simulink model "back_left_leg_assembly"  (R2023b)
settings: Solver=VariableStepAuto  StartTime=0.0  StopTime=10.0  RelTol=1e-3  AbsTol=1e-3  EnableMultiTasking=on
undefined symbols (not defined in the file): robot_conversions, robot_joints, robot_weights, X, Y, Z
libraries: sm_lib x17, nesl_utility x7, cstblocks x6, simulink x3, simulink_extras x3
settings Model: Creator=ivano  LastModifiedBy=ivano
settings SolverCC: AutoScaleAbsTol=off  AlgebraicLoopSolver=TrustRegion  MaxZcPerStep=1
settings DataIOCC: LimitDataPoints=on  MaxDataPoints=10000
settings OptimizationCC: ReuseModelBlockBuffer=off  LifeSpan=inf
settings DebuggingCC: UnconnectedInputMsg=warning  UnconnectedOutputMsg=warning  UnconnectedLineMsg=warning  AllowSymbolicDim=off  SubsystemReferenceDiagnosticForUnitTest=warning  SFUnexpectedBacktrackingDiag=warning  SFNoUnconditionalDefaultTransitionDiag=warning  SFExecutionAtInitializationDiag=none  ArithmeticOperatorsInVariantConditions=warning
settings ModelReferenceCC: EnableRefExpFcnMdlSchedulingChecks=on
settings SFSimCC: SimUseLocalCustomCode=off  CustomCodeUndefinedFunction=UseInterfaceOnly
settings RTWCC: RTWUseLocalCustomCode=off  DLArmComputeVersion=19.05
settings CodeAppCC: StateflowObjectComments=on
settings GRTTargetCC: TargetLangStandard=C89/C90 (ANSI)
settings ConfigComp: CovMetricSettings=dw  CovSaveCumulativeToWorkspaceVar=on  CovSaveSingleToWorkspaceVar=on  CovExternalEMLEnable=off  CovSFcnEnable=off
settings SimscapeCC: SimscapeLogType=all  SimscapeLogSimulationStatistics=on  SimscapeLogDataHistory=10000

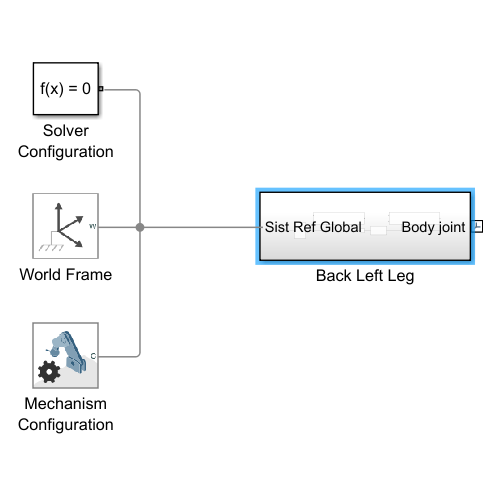
[thumbnail: Simulink's stored preview of the top-level diagram]
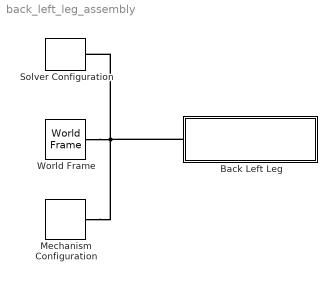
== system back_left_leg_assembly ==
  Back Left Leg : Subsystem
  Mechanism Configuration : sm_lib/Utilities/Mechanism Configuration  UniformGravity=Constant  GravityVector=[0 0 -9.80665]  GravityVectorUnits=m/s^2  LinearizationDelta=0.001  JointModeTransitionNonlinearIterations=2
  Solver Configuration : nesl_utility/Solver Configuration  PhysicalDomain=network_engine_domain  SubClassName=solver  LeftPortType=input  RightPortType=generic  Tones=[]  Harmonics=[]  SimulateNoise=off  Profile=off  UseLocalSampling=off  EnableSwitchedLinearOptims=on  FrequencyDomain=off  UseCCode=off  RelTol=0.001  AbsTol=1e-06  MinStep=1e-09  ToWorkspace=off  RevertToSquareIcSolve=off  NumHomotopyIterations=100  PhasorMode=off  PhasorModeNumHarmonics=1  ConsistencySolver=NEWTON_XTOL_AFTER_FTOL  IndexReductionMethod=DerivativeReplacement  DoDC=off  ResidualTolerance=1e-09  ConsistencyTolSource=GLOBAL  ConsistencyAbsTol=0.001  ConsistencyRelTol=0.001  ConsistencyTolFactor=0.001  UseLocalSolver=off  LocalSolverChoice=NE_BACKWARD_EULER_ADVANCER  ResolveIndetEquations=on  FunctionEvalNumThread=1  LocalSolverSampleTime=0.001  DoFixedCost=off  MaxNonlinIter=3  MaxModeIter=2  ComputeImpulses=off  ImpulseIterations=2  LinearAlgebra=Sparse  LinearAlgebraNumThread=0  EquationFormulation=NE_TIME_EF  DelaysMemoryBudget=1024  AutomaticFiltering=on  FilteringTimeConstant=0.001  PartitionStorageMethod=AS_NEEDED  PartitionMemoryBudget=1024  PartitionMethod=FAST  MultibodyUseLocalSolver=off  MultibodyLocalSolverChoice=ODE1  MultibodyLocalSolverSampleTime=0.001
  World Frame : sm_lib/Frames and Transforms/World Frame
  connections:
  World Frame/RConn1 -- Mechanism Configuration/RConn1 -- Back Left Leg/LConn1 -- Solver Configuration/RConn1

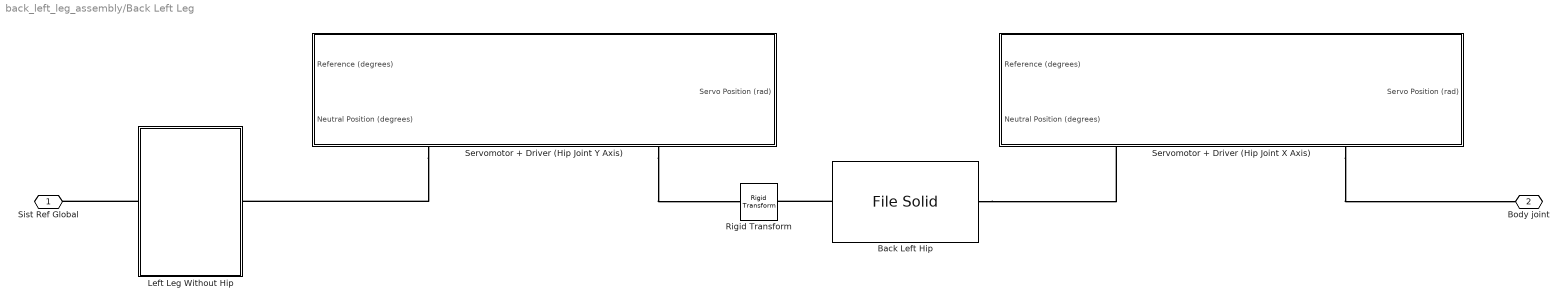
== system back_left_leg_assembly/Back Left Leg ==
  Back Left Hip : sm_lib/Body Elements/File Solid  ExtGeomFileName=..\3D Models\Hip\STEP Simscape Models\hip_bl.step  UnitType=FromFile  ExtGeomFileUnits=m  StepReaderType=HEX  ExportConvexHullGeometry=off  InertiaType=CalculateFromGeometry  Mass=robot_weights.hip  MassUnits=g  CenterOfMass=[0 0 0]  CenterOfMassUnits=m  MomentsOfInertia=[1 1 1]  MomentsOfInertiaUnits=kg*m^2  ProductsOfInertia=[0 0 0]  ProductsOfInertiaUnits=kg*m^2  BasedOnType=Mass  Density=1000  DensityUnits=kg/m^3  DoExposeReferenceFrame=off  SerializedFrames=<Frames><Frame><Id>Frame1</Id><Value><Name>Femur_joint</Name><Origin><Source>GeometricFeature</Source><FeatureName>circular curve 60</FeatureName></Origin><PrimaryAxis><DefinedDirection>+Z</DefinedDirection><Source>ReferenceFrame</Source><SourceDirection>+Z</SourceDirection><FeatureName></FeatureName></PrimaryAxis><SecondaryAxis><DefinedDirection>+X</DefinedDirection><Source>ReferenceFrame</Source><SourceDirection>+X</SourceDirection><FeatureName></FeatureName></SecondaryAxis></Value></Frame><Frame><Id>Frame2</Id><Value><Name>Body_joint</Name><Origin><Source>GeometricFeature</Source><FeatureName>circular curve 72</FeatureName></Origin><PrimaryAxis><DefinedDirection>+Z</DefinedDirection><Source>ReferenceFrame</Source><SourceDirection>+Z</SourceDirection><FeatureName></FeatureName></PrimaryAxis><SecondaryAxis><DefinedDirection>+X</DefinedDirection><Source>ReferenceFrame</Source><SourceDirection>+X</SourceDirection><FeatureName></FeatureName></SecondaryAxis></Value></Frame></Frames>  GraphicType=FromGeometry  MarkerShape=Sphere  MarkerSize=10  GraphicVisPropType=SimpleVisualProperties  GraphicDiffuseColor=[0.5 0.5 0.5]  GraphicSpecularColor=[0.5 0.5 0.5 1.0]  GraphicAmbientColor=[0.15 0.15 0.15 1.0]  GraphicEmissiveColor=[0.0 0.0 0.0 1.0]  GraphicShininess=75  GraphicOpacity=1.0
  Left Leg Without Hip : Subsystem
  Rigid Transform : sm_lib/Frames and Transforms/Rigid Transform  TranslationMethod=Cartesian  TranslationStandardOffset=0  TranslationStandardOffsetUnits=m  TranslationStandardAxis=+Z  TranslationCartesianOffset=[0 9.477 0]  TranslationCartesianOffsetUnits=mm  TranslationROffset=0  TranslationROffsetUnits=m  TranslationZOffset=0  TranslationZOffsetUnits=m  TranslationThetaOffset=0  TranslationThetaOffsetUnits=deg  RotationMethod=None  RotationAngleUnits=deg  RotationStandardAxis=+Z  RotationAngle=0.0  RotationArbitraryAxis=[0 0 1]  FollAlignAxisA=+X  BaseAlignAxisA=+Y  FollAlignAxisB=+Y  BaseAlignAxisB=+Z  RotationSequenceAxes=FollowerAxes  RotationSequence=XYX  RotationSequenceAngles=[0 0 0]  RotationSequenceAnglesUnits=deg  RotationMatrix=[1 0 0; 0 1 0; 0 0 1]  Quaternion=[1 0 0 0]
  Servomotor + Driver (Hip Joint X Axis) : Subsystem
      settings: PortSchema="{\"entries\":[{\"content\":{\"sides\":[{\"content\":{\"connectorIds\":[\"In1\",\"In2\"]},\"type\":\"ConnectorPlacement.EquallySpacedRectSide\",\"uuid\":\"34aed934-2639-4a00-aaee-cf3027466446\"},{\"content\":{\"connectorIds\":[\"Out1\"],\"side\":\"RIGHT\"},\"type\":\"ConnectorPlacement.EquallySpacedRectSide\",\"uuid\":\"6801890d-3466-4e37-90e8-6d1471e5b2c4\"},{\"content\":{\"side\":\"TOP\"},\"type\":\"ConnectorPlacement.EquallySpacedRectSide\",\"uuid\":\"bc3191aa-eca4-4e32-9fcf-8d5b7059b0b6\"},{\"content\":{\"connectorIds\":[\"RConn1\",\"RConn2\"],\"side\":\"BOTTOM\"},\"type\":\"ConnectorPlacement.EquallySpacedRectSide\",\"uuid\":\"867f09f9-bc2c-4353-bf05-5e7fc6d76fc7\"}]},\"type\":\"ConnectorPlacement.EquallySpacedConnector\",\"uuid\":\"7616468a-464c-41b8-bfd7-188201b948eb\"}],\"packageUris\":[\"http://schema.mathworks.com/mf0/Connector/R2020b\"],\"version\":\"1.0\"}"
  Servomotor + Driver (Hip Joint Y Axis) : Subsystem
      settings: PortSchema="{\"entries\":[{\"content\":{\"sides\":[{\"content\":{\"connectorIds\":[\"In1\",\"In2\"]},\"type\":\"ConnectorPlacement.EquallySpacedRectSide\",\"uuid\":\"34aed934-2639-4a00-aaee-cf3027466446\"},{\"content\":{\"connectorIds\":[\"Out1\"],\"side\":\"RIGHT\"},\"type\":\"ConnectorPlacement.EquallySpacedRectSide\",\"uuid\":\"6801890d-3466-4e37-90e8-6d1471e5b2c4\"},{\"content\":{\"side\":\"TOP\"},\"type\":\"ConnectorPlacement.EquallySpacedRectSide\",\"uuid\":\"bc3191aa-eca4-4e32-9fcf-8d5b7059b0b6\"},{\"content\":{\"connectorIds\":[\"RConn1\",\"RConn2\"],\"side\":\"BOTTOM\"},\"type\":\"ConnectorPlacement.EquallySpacedRectSide\",\"uuid\":\"867f09f9-bc2c-4353-bf05-5e7fc6d76fc7\"}]},\"type\":\"ConnectorPlacement.EquallySpacedConnector\",\"uuid\":\"7616468a-464c-41b8-bfd7-188201b948eb\"}],\"packageUris\":[\"http://schema.mathworks.com/mf0/Connector/R2020b\"],\"version\":\"1.0\"}"
  Sist Ref Global : PMIOPort  Side=Left
  Body joint : PMIOPort  Port=2  Side=Right
  connections:
  Servomotor + Driver (Hip Joint Y Axis)/RConn2 -- Rigid Transform/RConn1
  Back Left Hip/LConn1 -- Rigid Transform/LConn1
  Servomotor + Driver (Hip Joint Y Axis)/RConn1 -- Left Leg Without Hip/RConn1
  Left Leg Without Hip/LConn1 -- Sist Ref Global/RConn1
  Back Left Hip/RConn1 -- Servomotor + Driver (Hip Joint X Axis)/RConn1
  Servomotor + Driver (Hip Joint X Axis)/RConn2 -- Body joint/RConn1

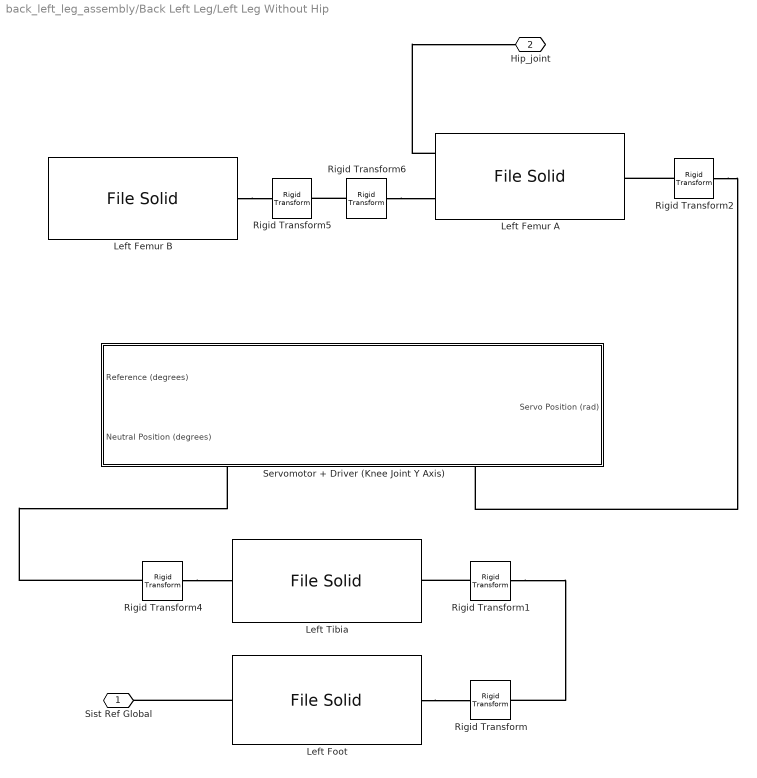
== system back_left_leg_assembly/Back Left Leg/Left Leg Without Hip ==
  Left Femur A : sm_lib/Body Elements/File Solid  ExtGeomFileName=..\3D Models\Femur\STEP Simscape Models\femur_l_a.step  UnitType=FromFile  ExtGeomFileUnits=m  StepReaderType=HEX  ExportConvexHullGeometry=off  InertiaType=CalculateFromGeometry  Mass=robot_weights.femur_a  MassUnits=g  CenterOfMass=[0 0 0]  CenterOfMassUnits=m  MomentsOfInertia=[1 1 1]  MomentsOfInertiaUnits=kg*m^2  ProductsOfInertia=[0 0 0]  ProductsOfInertiaUnits=kg*m^2  BasedOnType=Mass  Density=1000  DensityUnits=kg/m^3  DoExposeReferenceFrame=off  SerializedFrames=<Frames><Frame><Id>Frame1</Id><Value><Name>Hip_joint</Name><Origin><Source>GeometricFeature</Source><FeatureName>circular curve 110</FeatureName></Origin><PrimaryAxis><DefinedDirection>+Z</DefinedDirection><Source>ReferenceFrame</Source><SourceDirection>+Z</SourceDirection><FeatureName></FeatureName></PrimaryAxis><SecondaryAxis><DefinedDirection>+X</DefinedDirection><Source>ReferenceFrame</Source><SourceDirection>+X</SourceDirection><FeatureName></FeatureName></SecondaryAxis></Value></Frame><Frame><Id>Frame2</Id><Value><Name>Tibia_joint</Name><Origin><Source>GeometricFeature</Source><FeatureName>circular curve 126</FeatureName></Origin><PrimaryAxis><DefinedDirection>+Z</DefinedDirection><Source>ReferenceFrame</Source><SourceDirection>+Z</SourceDirection><FeatureName></FeatureName></PrimaryAxis><SecondaryAxis><DefinedDirection>+X</DefinedDirection><Source>ReferenceFrame</Source><SourceDirection>+X</SourceDirection><FeatureName></FeatureName></SecondaryAxis></Value></Frame><Frame><Id>Frame3</Id><Value><Name>Femur_B_joint</Name><Origin><Source>GeometricFeature</Source><FeatureName>circular curve 10</FeatureName></Origin><PrimaryAxis><DefinedDirection>+Z</DefinedDirection><Source>ReferenceFrame</Source><SourceDirection>+Z</SourceDirection><FeatureName></FeatureName></PrimaryAxis><SecondaryAxis><DefinedDirection>+X</DefinedDirection><Source>ReferenceFrame</Source><SourceDirection>+X</SourceDirection><FeatureName></FeatureName></SecondaryAxis></Value></Frame></Frames>  GraphicType=FromGeometry  MarkerShape=Sphere  MarkerSize=10  GraphicVisPropType=SimpleVisualProperties  GraphicDiffuseColor=[0.5 0.5 0.5]  GraphicSpecularColor=[0.5 0.5 0.5 1.0]  GraphicAmbientColor=[0.15 0.15 0.15 1.0]  GraphicEmissiveColor=[0.0 0.0 0.0 1.0]  GraphicShininess=75  GraphicOpacity=1.0
  Left Femur B : sm_lib/Body Elements/File Solid  ExtGeomFileName=..\3D Models\Femur\STEP Simscape Models\femur_l_b.step  UnitType=FromFile  ExtGeomFileUnits=m  StepReaderType=HEX  ExportConvexHullGeometry=off  InertiaType=CalculateFromGeometry  Mass=robot_weights.femur_b  MassUnits=g  CenterOfMass=[0 0 0]  CenterOfMassUnits=m  MomentsOfInertia=[1 1 1]  MomentsOfInertiaUnits=kg*m^2  ProductsOfInertia=[0 0 0]  ProductsOfInertiaUnits=kg*m^2  BasedOnType=Mass  Density=1000  DensityUnits=kg/m^3  DoExposeReferenceFrame=off  SerializedFrames=<Frames><Frame><Id>Frame1</Id><Value><Name>Femur_A_joint</Name><Origin><Source>GeometricFeature</Source><FeatureName>circular curve 235</FeatureName></Origin><PrimaryAxis><DefinedDirection>+Z</DefinedDirection><Source>ReferenceFrame</Source><SourceDirection>+Z</SourceDirection><FeatureName></FeatureName></PrimaryAxis><SecondaryAxis><DefinedDirection>+X</DefinedDirection><Source>ReferenceFrame</Source><SourceDirection>+X</SourceDirection><FeatureName></FeatureName></SecondaryAxis></Value></Frame></Frames>  GraphicType=FromGeometry  MarkerShape=Sphere  MarkerSize=10  GraphicVisPropType=SimpleVisualProperties  GraphicDiffuseColor=[0.5 0.5 0.5]  GraphicSpecularColor=[0.5 0.5 0.5 1.0]  GraphicAmbientColor=[0.15 0.15 0.15 1.0]  GraphicEmissiveColor=[0.0 0.0 0.0 1.0]  GraphicShininess=75  GraphicOpacity=1.0
  Left Foot : sm_lib/Body Elements/File Solid  ExtGeomFileName=..\3D Models\Feet\STEP Simscape Models\foot_l.step  UnitType=FromFile  ExtGeomFileUnits=m  StepReaderType=HEX  ExportConvexHullGeometry=off  InertiaType=CalculateFromGeometry  Mass=robot_weights.foot  MassUnits=g  CenterOfMass=[0 0 0]  CenterOfMassUnits=m  MomentsOfInertia=[1 1 1]  MomentsOfInertiaUnits=kg*m^2  ProductsOfInertia=[0 0 0]  ProductsOfInertiaUnits=kg*m^2  BasedOnType=Mass  Density=1000  DensityUnits=kg/m^3  DoExposeReferenceFrame=on  SerializedFrames=<Frames><Frame><Id>Frame1</Id><Value><Name>Tibia_joint</Name><Origin><Source>GeometricFeature</Source><FeatureName>circular curve 17</FeatureName></Origin><PrimaryAxis><DefinedDirection>+Z</DefinedDirection><Source>ReferenceFrame</Source><SourceDirection>+Z</SourceDirection><FeatureName></FeatureName></PrimaryAxis><SecondaryAxis><DefinedDirection>+X</DefinedDirection><Source>ReferenceFrame</Source><SourceDirection>+X</SourceDirection><FeatureName></FeatureName></SecondaryAxis></Value></Frame></Frames>  GraphicType=FromGeometry  MarkerShape=Sphere  MarkerSize=10  GraphicVisPropType=SimpleVisualProperties  GraphicDiffuseColor=[0.5 0.5 0.5]  GraphicSpecularColor=[0.5 0.5 0.5 1.0]  GraphicAmbientColor=[0.15 0.15 0.15 1.0]  GraphicEmissiveColor=[0.0 0.0 0.0 1.0]  GraphicShininess=75  GraphicOpacity=1.0
  Left Tibia : sm_lib/Body Elements/File Solid  ExtGeomFileName=..\3D Models\Tibia\STEP Simscape Models\tibia_l.step  UnitType=FromFile  ExtGeomFileUnits=m  StepReaderType=HEX  ExportConvexHullGeometry=off  InertiaType=CalculateFromGeometry  Mass=robot_weights.tibia  MassUnits=g  CenterOfMass=[0 0 0]  CenterOfMassUnits=m  MomentsOfInertia=[1 1 1]  MomentsOfInertiaUnits=kg*m^2  ProductsOfInertia=[0 0 0]  ProductsOfInertiaUnits=kg*m^2  BasedOnType=Mass  Density=1000  DensityUnits=kg/m^3  DoExposeReferenceFrame=off  SerializedFrames=<Frames><Frame><Id>Frame1</Id><Value><Name>Foot_joint</Name><Origin><Source>GeometricFeature</Source><FeatureName>circular curve 168</FeatureName></Origin><PrimaryAxis><DefinedDirection>+Z</DefinedDirection><Source>ReferenceFrame</Source><SourceDirection>+Z</SourceDirection><FeatureName></FeatureName></PrimaryAxis><SecondaryAxis><DefinedDirection>+X</DefinedDirection><Source>ReferenceFrame</Source><SourceDirection>+X</SourceDirection><FeatureName></FeatureName></SecondaryAxis></Value></Frame><Frame><Id>Frame2</Id><Value><Name>Femur_A_joint</Name><Origin><Source>GeometricFeature</Source><FeatureName>circular curve 170</FeatureName></Origin><PrimaryAxis><DefinedDirection>+Z</DefinedDirection><Source>ReferenceFrame</Source><SourceDirection>+Z</SourceDirection><FeatureName></FeatureName></PrimaryAxis><SecondaryAxis><DefinedDirection>+X</DefinedDirection><Source>ReferenceFrame</Source><SourceDirection>+X</SourceDirection><FeatureName></FeatureName></SecondaryAxis></Value></Frame></Frames>  GraphicType=FromGeometry  MarkerShape=Sphere  MarkerSize=10  GraphicVisPropType=SimpleVisualProperties  GraphicDiffuseColor=[0.5 0.5 0.5]  GraphicSpecularColor=[0.5 0.5 0.5 1.0]  GraphicAmbientColor=[0.15 0.15 0.15 1.0]  GraphicEmissiveColor=[0.0 0.0 0.0 1.0]  GraphicShininess=75  GraphicOpacity=1.0
  Rigid Transform : sm_lib/Frames and Transforms/Rigid Transform  TranslationMethod=Cartesian  TranslationStandardOffset=0  TranslationStandardOffsetUnits=m  TranslationStandardAxis=+Z  TranslationCartesianOffset=[0 -4.826/2 0]  TranslationCartesianOffsetUnits=mm  TranslationROffset=0  TranslationROffsetUnits=m  TranslationZOffset=0  TranslationZOffsetUnits=m  TranslationThetaOffset=0  TranslationThetaOffsetUnits=deg  RotationMethod=None  RotationAngleUnits=deg  RotationStandardAxis=+Z  RotationAngle=0.0  RotationArbitraryAxis=[0 0 1]  FollAlignAxisA=+X  BaseAlignAxisA=+Y  FollAlignAxisB=+Y  BaseAlignAxisB=+Z  RotationSequenceAxes=FollowerAxes  RotationSequence=XYX  RotationSequenceAngles=[0 0 0]  RotationSequenceAnglesUnits=deg  RotationMatrix=[1 0 0; 0 1 0; 0 0 1]  Quaternion=[1 0 0 0]
  Rigid Transform1 : sm_lib/Frames and Transforms/Rigid Transform  TranslationMethod=Cartesian  TranslationStandardOffset=0  TranslationStandardOffsetUnits=m  TranslationStandardAxis=+Z  TranslationCartesianOffset=[0 4.207/2 0]  TranslationCartesianOffsetUnits=mm  TranslationROffset=0  TranslationROffsetUnits=m  TranslationZOffset=0  TranslationZOffsetUnits=m  TranslationThetaOffset=0  TranslationThetaOffsetUnits=deg  RotationMethod=None  RotationAngleUnits=deg  RotationStandardAxis=+Z  RotationAngle=0.0  RotationArbitraryAxis=[0 0 1]  FollAlignAxisA=+X  BaseAlignAxisA=+Y  FollAlignAxisB=+Y  BaseAlignAxisB=+Z  RotationSequenceAxes=FollowerAxes  RotationSequence=XYX  RotationSequenceAngles=[0 0 0]  RotationSequenceAnglesUnits=deg  RotationMatrix=[1 0 0; 0 1 0; 0 0 1]  Quaternion=[1 0 0 0]
  Rigid Transform{2,4..6} (4 alike) : sm_lib/Frames and Transforms/Rigid Transform  TranslationMethod=Cartesian  TranslationStandardOffset=0  TranslationStandardOffsetUnits=m  TranslationStandardAxis=+Z  TranslationCartesianOffset=[0 -21.448/2 0]  TranslationCartesianOffsetUnits=mm  TranslationROffset=0  TranslationROffsetUnits=m  TranslationZOffset=0  TranslationZOffsetUnits=m  TranslationThetaOffset=0  TranslationThetaOffsetUnits=deg  RotationMethod=None  RotationAngleUnits=deg  RotationStandardAxis=+Z  RotationAngle=0.0  RotationArbitraryAxis=[0 0 1]  FollAlignAxisA=+X  BaseAlignAxisA=+Y  FollAlignAxisB=+Y  BaseAlignAxisB=+Z  RotationSequenceAxes=FollowerAxes  RotationSequence=XYX  RotationSequenceAngles=[0 0 0]  RotationSequenceAnglesUnits=deg  RotationMatrix=[1 0 0; 0 1 0; 0 0 1]  Quaternion=[1 0 0 0]
  Servomotor + Driver (Knee Joint Y Axis) : Subsystem
      settings: PortSchema="{\"entries\":[{\"content\":{\"sides\":[{\"content\":{\"connectorIds\":[\"In1\",\"In2\"]},\"type\":\"ConnectorPlacement.EquallySpacedRectSide\",\"uuid\":\"34aed934-2639-4a00-aaee-cf3027466446\"},{\"content\":{\"connectorIds\":[\"Out1\"],\"side\":\"RIGHT\"},\"type\":\"ConnectorPlacement.EquallySpacedRectSide\",\"uuid\":\"6801890d-3466-4e37-90e8-6d1471e5b2c4\"},{\"content\":{\"side\":\"TOP\"},\"type\":\"ConnectorPlacement.EquallySpacedRectSide\",\"uuid\":\"bc3191aa-eca4-4e32-9fcf-8d5b7059b0b6\"},{\"content\":{\"connectorIds\":[\"RConn1\",\"RConn2\"],\"side\":\"BOTTOM\"},\"type\":\"ConnectorPlacement.EquallySpacedRectSide\",\"uuid\":\"867f09f9-bc2c-4353-bf05-5e7fc6d76fc7\"}]},\"type\":\"ConnectorPlacement.EquallySpacedConnector\",\"uuid\":\"7616468a-464c-41b8-bfd7-188201b948eb\"}],\"packageUris\":[\"http://schema.mathworks.com/mf0/Connector/R2020b\"],\"version\":\"1.0\"}"
  Sist Ref Global : PMIOPort  Side=Left
  Hip_joint : PMIOPort  Port=2  Side=Right
  connections:
  Rigid Transform1/LConn1 -- Left Tibia/LConn1
  Rigid Transform1/RConn1 -- Rigid Transform/RConn1
  Left Foot/LConn1 -- Rigid Transform/LConn1
  Rigid Transform2/LConn1 -- Left Femur A/RConn1
  Rigid Transform4/RConn1 -- Servomotor + Driver (Knee Joint Y Axis)/RConn1
  Rigid Transform4/LConn1 -- Left Tibia/RConn1
  Left Foot/RConn1 -- Sist Ref Global/RConn1
  Left Femur B/LConn1 -- Rigid Transform5/LConn1
  Rigid Transform6/RConn1 -- Rigid Transform5/RConn1
  Rigid Transform2/RConn1 -- Servomotor + Driver (Knee Joint Y Axis)/RConn2
  Rigid Transform6/LConn1 -- Left Femur A/LConn2
  Left Femur A/LConn1 -- Hip_joint/RConn1

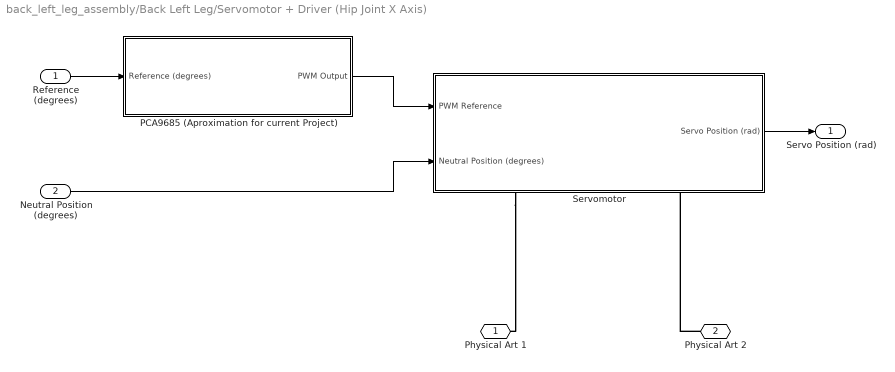
== system back_left_leg_assembly/Back Left Leg/Servomotor + Driver (Hip Joint X Axis) ==
  Reference (degrees) : Inport
  Neutral Position (degrees) : Inport  Port=2
  PCA9685 (Aproximation for current Project) : Subsystem
  Servomotor : Subsystem
      settings: PortSchema="{\"entries\":[{\"content\":{\"sides\":[{\"content\":{\"connectorIds\":[\"In1\",\"In2\"]},\"type\":\"ConnectorPlacement.EquallySpacedRectSide\",\"uuid\":\"eeff66d3-7cb0-4fe9-90b5-92935711e170\"},{\"content\":{\"connectorIds\":[\"Out1\"],\"side\":\"RIGHT\"},\"type\":\"ConnectorPlacement.EquallySpacedRectSide\",\"uuid\":\"4c1729b3-3224-4ed4-9eed-359312bd5e7e\"},{\"content\":{\"side\":\"TOP\"},\"type\":\"ConnectorPlacement.EquallySpacedRectSide\",\"uuid\":\"ee6ed6e9-0c82-482d-bf53-5898b89012ab\"},{\"content\":{\"connectorIds\":[\"RConn1\",\"RConn2\"],\"side\":\"BOTTOM\"},\"type\":\"ConnectorPlacement.EquallySpacedRectSide\",\"uuid\":\"6da00c0c-ced6-4450-8de1-d587d7c692e9\"}]},\"type\":\"ConnectorPlacement.EquallySpacedConnector\",\"uuid\":\"38b9234f-cec7-4245-8a78-4426dc0791bf\"}],\"packageUris\":[\"http://schema.mathworks.com/mf0/Connector/R2020b\"],\"version\":\"1.0\"}"
  Physical Art 1 : PMIOPort  Side=Right
  Physical Art 2 : PMIOPort  Port=2  Side=Right
  Servo Position (rad) : Outport
  wires:
  PCA9685 (Aproximation for current Project)/1(PWM Output) -> Servomotor/1(PWM Reference)
  Neutral Position (degrees)/1 -> Servomotor/2(Neutral Position (degrees))
  Reference (degrees)/1 -> PCA9685 (Aproximation for current Project)/1(Reference (degrees))
  Servomotor/1(Servo Position (rad)) -> Servo Position (rad)/1
  connections:
  Servomotor/RConn1 -- Physical Art 1/RConn1
  Physical Art 2/RConn1 -- Servomotor/RConn2

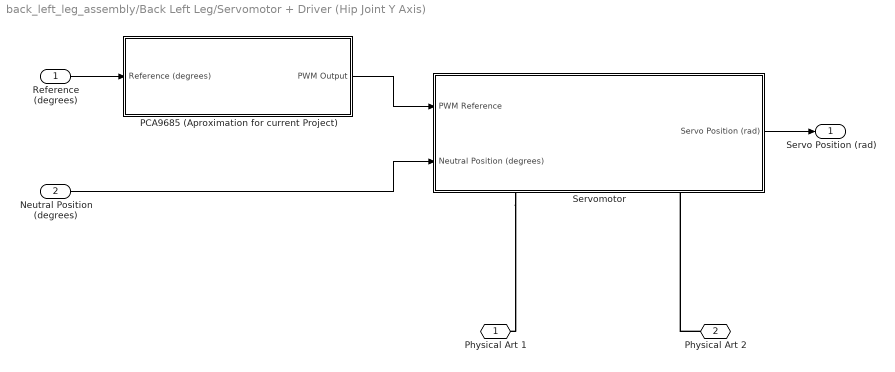
== system back_left_leg_assembly/Back Left Leg/Servomotor + Driver (Hip Joint Y Axis) ==
  Reference (degrees) : Inport
  Neutral Position (degrees) : Inport  Port=2
  PCA9685 (Aproximation for current Project) : Subsystem
  Servomotor : Subsystem
      settings: PortSchema="{\"entries\":[{\"content\":{\"sides\":[{\"content\":{\"connectorIds\":[\"In1\",\"In2\"]},\"type\":\"ConnectorPlacement.EquallySpacedRectSide\",\"uuid\":\"eeff66d3-7cb0-4fe9-90b5-92935711e170\"},{\"content\":{\"connectorIds\":[\"Out1\"],\"side\":\"RIGHT\"},\"type\":\"ConnectorPlacement.EquallySpacedRectSide\",\"uuid\":\"4c1729b3-3224-4ed4-9eed-359312bd5e7e\"},{\"content\":{\"side\":\"TOP\"},\"type\":\"ConnectorPlacement.EquallySpacedRectSide\",\"uuid\":\"ee6ed6e9-0c82-482d-bf53-5898b89012ab\"},{\"content\":{\"connectorIds\":[\"RConn1\",\"RConn2\"],\"side\":\"BOTTOM\"},\"type\":\"ConnectorPlacement.EquallySpacedRectSide\",\"uuid\":\"6da00c0c-ced6-4450-8de1-d587d7c692e9\"}]},\"type\":\"ConnectorPlacement.EquallySpacedConnector\",\"uuid\":\"38b9234f-cec7-4245-8a78-4426dc0791bf\"}],\"packageUris\":[\"http://schema.mathworks.com/mf0/Connector/R2020b\"],\"version\":\"1.0\"}"
  Physical Art 1 : PMIOPort  Side=Right
  Physical Art 2 : PMIOPort  Port=2  Side=Right
  Servo Position (rad) : Outport
  wires:
  PCA9685 (Aproximation for current Project)/1(PWM Output) -> Servomotor/1(PWM Reference)
  Neutral Position (degrees)/1 -> Servomotor/2(Neutral Position (degrees))
  Reference (degrees)/1 -> PCA9685 (Aproximation for current Project)/1(Reference (degrees))
  Servomotor/1(Servo Position (rad)) -> Servo Position (rad)/1
  connections:
  Servomotor/RConn1 -- Physical Art 1/RConn1
  Physical Art 2/RConn1 -- Servomotor/RConn2

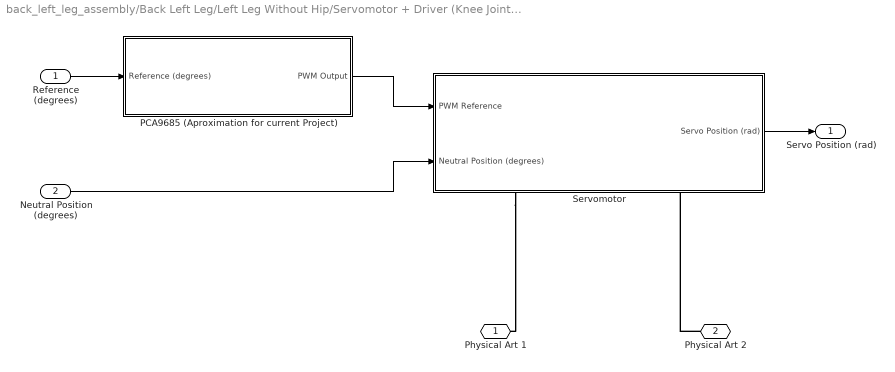
== system back_left_leg_assembly/Back Left Leg/Left Leg Without Hip/Servomotor + Driver (Knee Joint Y Axis) ==
  Reference (degrees) : Inport
  Neutral Position (degrees) : Inport  Port=2
  PCA9685 (Aproximation for current Project) : Subsystem
  Servomotor : Subsystem
      settings: PortSchema="{\"entries\":[{\"content\":{\"sides\":[{\"content\":{\"connectorIds\":[\"In1\",\"In2\"]},\"type\":\"ConnectorPlacement.EquallySpacedRectSide\",\"uuid\":\"eeff66d3-7cb0-4fe9-90b5-92935711e170\"},{\"content\":{\"connectorIds\":[\"Out1\"],\"side\":\"RIGHT\"},\"type\":\"ConnectorPlacement.EquallySpacedRectSide\",\"uuid\":\"4c1729b3-3224-4ed4-9eed-359312bd5e7e\"},{\"content\":{\"side\":\"TOP\"},\"type\":\"ConnectorPlacement.EquallySpacedRectSide\",\"uuid\":\"ee6ed6e9-0c82-482d-bf53-5898b89012ab\"},{\"content\":{\"connectorIds\":[\"RConn1\",\"RConn2\"],\"side\":\"BOTTOM\"},\"type\":\"ConnectorPlacement.EquallySpacedRectSide\",\"uuid\":\"6da00c0c-ced6-4450-8de1-d587d7c692e9\"}]},\"type\":\"ConnectorPlacement.EquallySpacedConnector\",\"uuid\":\"38b9234f-cec7-4245-8a78-4426dc0791bf\"}],\"packageUris\":[\"http://schema.mathworks.com/mf0/Connector/R2020b\"],\"version\":\"1.0\"}"
  Physical Art 1 : PMIOPort  Side=Right
  Physical Art 2 : PMIOPort  Port=2  Side=Right
  Servo Position (rad) : Outport
  wires:
  PCA9685 (Aproximation for current Project)/1(PWM Output) -> Servomotor/1(PWM Reference)
  Neutral Position (degrees)/1 -> Servomotor/2(Neutral Position (degrees))
  Reference (degrees)/1 -> PCA9685 (Aproximation for current Project)/1(Reference (degrees))
  Servomotor/1(Servo Position (rad)) -> Servo Position (rad)/1
  connections:
  Servomotor/RConn1 -- Physical Art 1/RConn1
  Physical Art 2/RConn1 -- Servomotor/RConn2

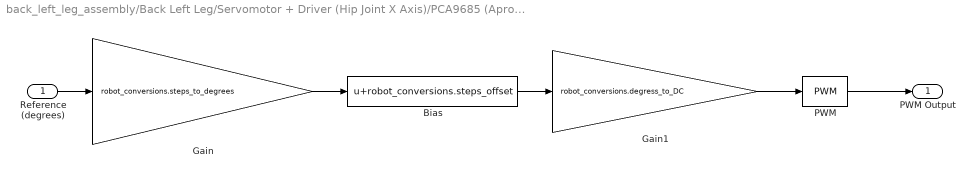
== system back_left_leg_assembly/Back Left Leg/Servomotor + Driver (Hip Joint X Axis)/PCA9685 (Aproximation for current Project) ==
  Reference (degrees) : Inport
  Bias : Bias  Bias=robot_conversions.steps_offset  SaturateOnIntegerOverflow=off
  Gain : Gain  Gain=robot_conversions.steps_to_degrees
  Gain1 : Gain  Gain=robot_conversions.degress_to_DC
  PWM : simulink/Discontinuities/PWM  DisableCoverage=on  Period=0.02  InitialDelay=0  DisallowZeroDutyCycle=off  RunAtFixedTimeIntervals=off  SampleTime=0.01
  PWM Output : Outport
  wires:
  Gain/1 -> Bias/1
  Bias/1 -> Gain1/1
  Gain1/1 -> PWM/1
  Reference (degrees)/1 -> Gain/1
  PWM/1 -> PWM Output/1

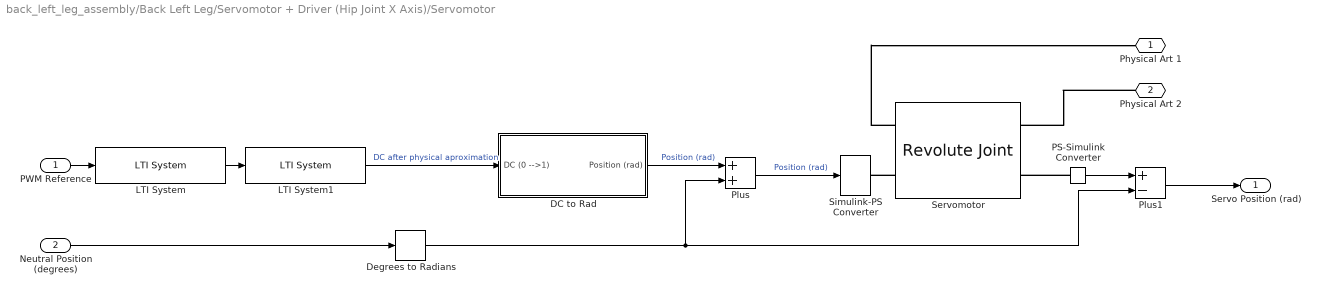
== system back_left_leg_assembly/Back Left Leg/Servomotor + Driver (Hip Joint X Axis)/Servomotor ==
  PWM Reference : Inport
  Neutral Position (degrees) : Inport  Port=2
  DC to Rad : Subsystem
  Degrees to Radians : simulink_extras/Transformations/Degrees to Radians
  LTI System : cstblocks/LTI System  sys=robot_tf.bessel_filter  IC=[]  PadeOrder=0
  LTI System1 : cstblocks/LTI System  sys=robot_tf.physical_tf  IC=[]  PadeOrder=0
  PS-Simulink Converter : nesl_utility/PS-Simulink Converter  PhysicalDomain=network_engine_domain  SubClassName=ps_output  LeftPortType=input  RightPortType=output  PseudoPeriodic=off  Frequencies=[]  VectorFormat=inherit  Unit=inherit  AffineConversion=off
  Plus : Sum
  Plus1 : Sum  Inputs=+-
  Servomotor : sm_lib/Joints/Revolute Joint  JointMode=Normal  SenseConstraintForce=off  SenseConstraintForceX=off  SenseConstraintForceY=off  SenseConstraintForceZ=off  SenseConstraintTorque=off  SenseConstraintTorqueX=off  SenseConstraintTorqueY=off  SenseConstraintTorqueZ=off  SenseTotalForce=off  SenseTotalForceX=off  SenseTotalForceY=off  SenseTotalForceZ=off  SenseTotalTorque=off  SenseTotalTorqueX=off  SenseTotalTorqueY=off  SenseTotalTorqueZ=off  CompositeWrenchDir=FollowerOnBase  CompositeWrenchFrame=BaseFrame  EquilibriumPosition=0  EquilibriumPositionUnits=rad  SpringStiffness=0  SpringStiffnessUnits=N*m/deg  DampingCoefficient=0  DampingCoefficientUnits=N*m/(deg/s)  TorqueActuationMode=ComputedTorque  MotionActuationMode=InputMotion  SensePosition=on  SenseVelocity=off  SenseAcceleration=off  SenseTorqueForce=off  SenseLowerLimitTorqueForce=off  SenseUpperLimitTorqueForce=off  LowerLimitSpecify=on  LowerLimitBound=robot_joints.q_limits(1)  LowerLimitBoundUnits=rad  LowerLimitStiffness=1e4  LowerLimitStiffnessUnits=N*m/deg  LowerLimitDamping=10  LowerLimitDampingUnits=N*m/(deg/s)  LowerLimitTransitionRegionWidth=0.1  LowerLimitTransitionRegionWidthUnits=deg  UpperLimitSpecify=on  UpperLimitBound=robot_joints.q_limits(2)  UpperLimitBoundUnits=rad  UpperLimitStiffness=1e4  UpperLimitStiffnessUnits=N*m/deg  UpperLimitDamping=10  UpperLimitDampingUnits=N*m/(deg/s)  UpperLimitTransitionRegionWidth=0.1  UpperLimitTransitionRegionWidthUnits=deg  PositionTargetSpecify=off  PositionTargetPriority=High  PositionTargetValue=0  PositionTargetValueUnits=deg  VelocityTargetSpecify=off  VelocityTargetPriority=High  VelocityTargetValue=0  VelocityTargetValueUnits=deg/s
  Simulink-PS Converter : nesl_utility/Simulink-PS Converter  PhysicalDomain=network_engine_domain  SubClassName=ps_input  LeftPortType=input  RightPortType=output  PseudoPeriodic=off  Frequencies=[]  NoiseDistribution=none  NoiseParameters=[]  Unit=1  AffineConversion=off  FilteringAndDerivatives=filter  SimscapeFilterOrder=2  InputFilterTimeConstant=0.001  UdotUserProvided=0
  Physical Art 1 : PMIOPort  Side=Right
  Physical Art 2 : PMIOPort  Port=2  Side=Right
  Servo Position (rad) : Outport
  wires:
  PWM Reference/1 -> LTI System/1
  LTI System/1 -> LTI System1/1
  LTI System1/1 -> DC to Rad/1(DC (0 -->1))  "DC after physical aproximation"
  Neutral Position (degrees)/1 -> Degrees to Radians/1
  DC to Rad/1(Position (rad)) -> Plus/1  "Position (rad)"
  Plus/1 -> Simulink-PS Converter/1  "Position (rad)"
  Degrees to Radians/1 -> Plus1/2, Plus/2
  PS-Simulink Converter/1 -> Plus1/1
  Plus1/1 -> Servo Position (rad)/1
  connections:
  PS-Simulink Converter/LConn1 -- Servomotor/RConn2
  Physical Art 2/RConn1 -- Servomotor/RConn1
  Servomotor/LConn1 -- Physical Art 1/RConn1
  Servomotor/LConn2 -- Simulink-PS Converter/RConn1

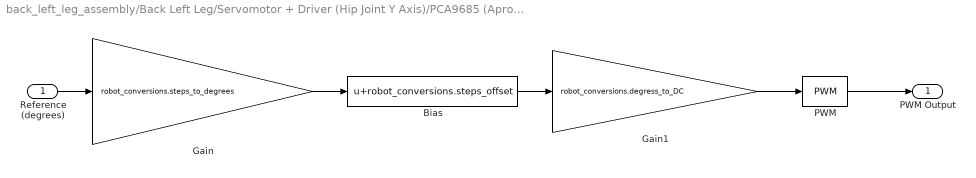
== system back_left_leg_assembly/Back Left Leg/Servomotor + Driver (Hip Joint Y Axis)/PCA9685 (Aproximation for current Project) ==
  Reference (degrees) : Inport
  Bias : Bias  Bias=robot_conversions.steps_offset  SaturateOnIntegerOverflow=off
  Gain : Gain  Gain=robot_conversions.steps_to_degrees
  Gain1 : Gain  Gain=robot_conversions.degress_to_DC
  PWM : simulink/Discontinuities/PWM  DisableCoverage=on  Period=0.02  InitialDelay=0  DisallowZeroDutyCycle=off  RunAtFixedTimeIntervals=off  SampleTime=0.01
  PWM Output : Outport
  wires:
  Gain/1 -> Bias/1
  Bias/1 -> Gain1/1
  Gain1/1 -> PWM/1
  Reference (degrees)/1 -> Gain/1
  PWM/1 -> PWM Output/1

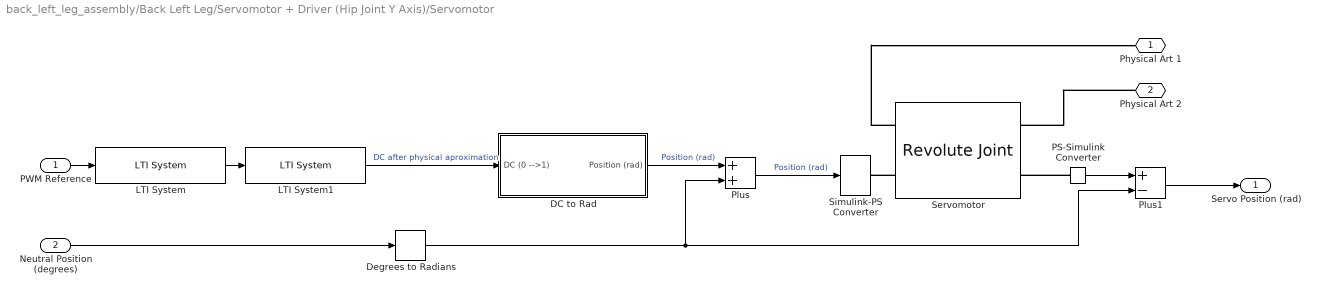
== system back_left_leg_assembly/Back Left Leg/Servomotor + Driver (Hip Joint Y Axis)/Servomotor ==
  PWM Reference : Inport
  Neutral Position (degrees) : Inport  Port=2
  DC to Rad : Subsystem
  Degrees to Radians : simulink_extras/Transformations/Degrees to Radians
  LTI System : cstblocks/LTI System  sys=robot_tf.bessel_filter  IC=[]  PadeOrder=0
  LTI System1 : cstblocks/LTI System  sys=robot_tf.physical_tf  IC=[]  PadeOrder=0
  PS-Simulink Converter : nesl_utility/PS-Simulink Converter  PhysicalDomain=network_engine_domain  SubClassName=ps_output  LeftPortType=input  RightPortType=output  PseudoPeriodic=off  Frequencies=[]  VectorFormat=inherit  Unit=inherit  AffineConversion=off
  Plus : Sum
  Plus1 : Sum  Inputs=+-
  Servomotor : sm_lib/Joints/Revolute Joint  JointMode=Normal  SenseConstraintForce=off  SenseConstraintForceX=off  SenseConstraintForceY=off  SenseConstraintForceZ=off  SenseConstraintTorque=off  SenseConstraintTorqueX=off  SenseConstraintTorqueY=off  SenseConstraintTorqueZ=off  SenseTotalForce=off  SenseTotalForceX=off  SenseTotalForceY=off  SenseTotalForceZ=off  SenseTotalTorque=off  SenseTotalTorqueX=off  SenseTotalTorqueY=off  SenseTotalTorqueZ=off  CompositeWrenchDir=FollowerOnBase  CompositeWrenchFrame=BaseFrame  EquilibriumPosition=0  EquilibriumPositionUnits=rad  SpringStiffness=0  SpringStiffnessUnits=N*m/deg  DampingCoefficient=0  DampingCoefficientUnits=N*m/(deg/s)  TorqueActuationMode=ComputedTorque  MotionActuationMode=InputMotion  SensePosition=on  SenseVelocity=off  SenseAcceleration=off  SenseTorqueForce=off  SenseLowerLimitTorqueForce=off  SenseUpperLimitTorqueForce=off  LowerLimitSpecify=on  LowerLimitBound=robot_joints.q_limits(1)  LowerLimitBoundUnits=rad  LowerLimitStiffness=1e4  LowerLimitStiffnessUnits=N*m/deg  LowerLimitDamping=10  LowerLimitDampingUnits=N*m/(deg/s)  LowerLimitTransitionRegionWidth=0.1  LowerLimitTransitionRegionWidthUnits=deg  UpperLimitSpecify=on  UpperLimitBound=robot_joints.q_limits(2)  UpperLimitBoundUnits=rad  UpperLimitStiffness=1e4  UpperLimitStiffnessUnits=N*m/deg  UpperLimitDamping=10  UpperLimitDampingUnits=N*m/(deg/s)  UpperLimitTransitionRegionWidth=0.1  UpperLimitTransitionRegionWidthUnits=deg  PositionTargetSpecify=off  PositionTargetPriority=High  PositionTargetValue=0  PositionTargetValueUnits=deg  VelocityTargetSpecify=off  VelocityTargetPriority=High  VelocityTargetValue=0  VelocityTargetValueUnits=deg/s
  Simulink-PS Converter : nesl_utility/Simulink-PS Converter  PhysicalDomain=network_engine_domain  SubClassName=ps_input  LeftPortType=input  RightPortType=output  PseudoPeriodic=off  Frequencies=[]  NoiseDistribution=none  NoiseParameters=[]  Unit=1  AffineConversion=off  FilteringAndDerivatives=filter  SimscapeFilterOrder=2  InputFilterTimeConstant=0.001  UdotUserProvided=0
  Physical Art 1 : PMIOPort  Side=Right
  Physical Art 2 : PMIOPort  Port=2  Side=Right
  Servo Position (rad) : Outport
  wires:
  PWM Reference/1 -> LTI System/1
  LTI System/1 -> LTI System1/1
  LTI System1/1 -> DC to Rad/1(DC (0 -->1))  "DC after physical aproximation"
  Neutral Position (degrees)/1 -> Degrees to Radians/1
  DC to Rad/1(Position (rad)) -> Plus/1  "Position (rad)"
  Plus/1 -> Simulink-PS Converter/1  "Position (rad)"
  Degrees to Radians/1 -> Plus1/2, Plus/2
  PS-Simulink Converter/1 -> Plus1/1
  Plus1/1 -> Servo Position (rad)/1
  connections:
  PS-Simulink Converter/LConn1 -- Servomotor/RConn2
  Physical Art 2/RConn1 -- Servomotor/RConn1
  Servomotor/LConn1 -- Physical Art 1/RConn1
  Servomotor/LConn2 -- Simulink-PS Converter/RConn1

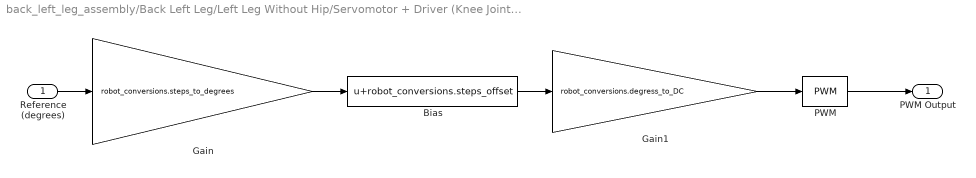
== system back_left_leg_assembly/Back Left Leg/Left Leg Without Hip/Servomotor + Driver (Knee Joint Y Axis)/PCA9685 (Aproximation for current Project) ==
  Reference (degrees) : Inport
  Bias : Bias  Bias=robot_conversions.steps_offset  SaturateOnIntegerOverflow=off
  Gain : Gain  Gain=robot_conversions.steps_to_degrees
  Gain1 : Gain  Gain=robot_conversions.degress_to_DC
  PWM : simulink/Discontinuities/PWM  DisableCoverage=on  Period=0.02  InitialDelay=0  DisallowZeroDutyCycle=off  RunAtFixedTimeIntervals=off  SampleTime=0.01
  PWM Output : Outport
  wires:
  Gain/1 -> Bias/1
  Bias/1 -> Gain1/1
  Gain1/1 -> PWM/1
  Reference (degrees)/1 -> Gain/1
  PWM/1 -> PWM Output/1

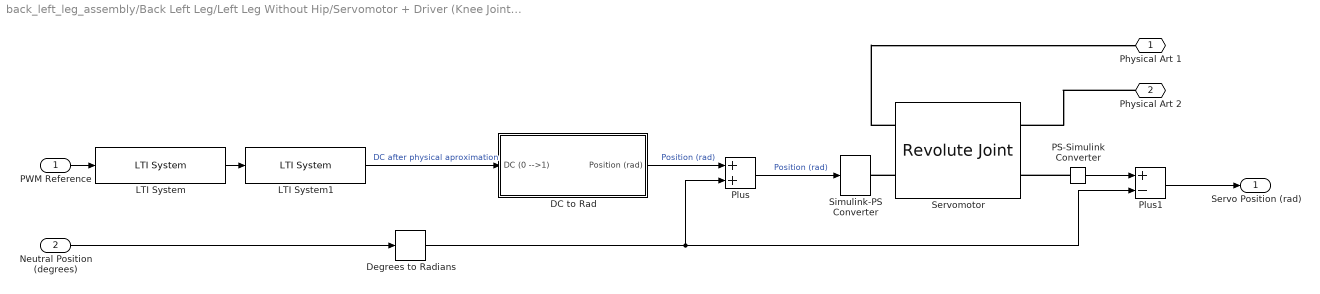
== system back_left_leg_assembly/Back Left Leg/Left Leg Without Hip/Servomotor + Driver (Knee Joint Y Axis)/Servomotor ==
  PWM Reference : Inport
  Neutral Position (degrees) : Inport  Port=2
  DC to Rad : Subsystem
  Degrees to Radians : simulink_extras/Transformations/Degrees to Radians
  LTI System : cstblocks/LTI System  sys=robot_tf.bessel_filter  IC=[]  PadeOrder=0
  LTI System1 : cstblocks/LTI System  sys=robot_tf.physical_tf  IC=[]  PadeOrder=0
  PS-Simulink Converter : nesl_utility/PS-Simulink Converter  PhysicalDomain=network_engine_domain  SubClassName=ps_output  LeftPortType=input  RightPortType=output  PseudoPeriodic=off  Frequencies=[]  VectorFormat=inherit  Unit=inherit  AffineConversion=off
  Plus : Sum
  Plus1 : Sum  Inputs=+-
  Servomotor : sm_lib/Joints/Revolute Joint  JointMode=Normal  SenseConstraintForce=off  SenseConstraintForceX=off  SenseConstraintForceY=off  SenseConstraintForceZ=off  SenseConstraintTorque=off  SenseConstraintTorqueX=off  SenseConstraintTorqueY=off  SenseConstraintTorqueZ=off  SenseTotalForce=off  SenseTotalForceX=off  SenseTotalForceY=off  SenseTotalForceZ=off  SenseTotalTorque=off  SenseTotalTorqueX=off  SenseTotalTorqueY=off  SenseTotalTorqueZ=off  CompositeWrenchDir=FollowerOnBase  CompositeWrenchFrame=BaseFrame  EquilibriumPosition=0  EquilibriumPositionUnits=rad  SpringStiffness=0  SpringStiffnessUnits=N*m/deg  DampingCoefficient=0  DampingCoefficientUnits=N*m/(deg/s)  TorqueActuationMode=ComputedTorque  MotionActuationMode=InputMotion  SensePosition=on  SenseVelocity=off  SenseAcceleration=off  SenseTorqueForce=off  SenseLowerLimitTorqueForce=off  SenseUpperLimitTorqueForce=off  LowerLimitSpecify=on  LowerLimitBound=robot_joints.q_limits(1)  LowerLimitBoundUnits=rad  LowerLimitStiffness=1e4  LowerLimitStiffnessUnits=N*m/deg  LowerLimitDamping=10  LowerLimitDampingUnits=N*m/(deg/s)  LowerLimitTransitionRegionWidth=0.1  LowerLimitTransitionRegionWidthUnits=deg  UpperLimitSpecify=on  UpperLimitBound=robot_joints.q_limits(2)  UpperLimitBoundUnits=rad  UpperLimitStiffness=1e4  UpperLimitStiffnessUnits=N*m/deg  UpperLimitDamping=10  UpperLimitDampingUnits=N*m/(deg/s)  UpperLimitTransitionRegionWidth=0.1  UpperLimitTransitionRegionWidthUnits=deg  PositionTargetSpecify=off  PositionTargetPriority=High  PositionTargetValue=0  PositionTargetValueUnits=deg  VelocityTargetSpecify=off  VelocityTargetPriority=High  VelocityTargetValue=0  VelocityTargetValueUnits=deg/s
  Simulink-PS Converter : nesl_utility/Simulink-PS Converter  PhysicalDomain=network_engine_domain  SubClassName=ps_input  LeftPortType=input  RightPortType=output  PseudoPeriodic=off  Frequencies=[]  NoiseDistribution=none  NoiseParameters=[]  Unit=1  AffineConversion=off  FilteringAndDerivatives=filter  SimscapeFilterOrder=2  InputFilterTimeConstant=0.001  UdotUserProvided=0
  Physical Art 1 : PMIOPort  Side=Right
  Physical Art 2 : PMIOPort  Port=2  Side=Right
  Servo Position (rad) : Outport
  wires:
  PWM Reference/1 -> LTI System/1
  LTI System/1 -> LTI System1/1
  LTI System1/1 -> DC to Rad/1(DC (0 -->1))  "DC after physical aproximation"
  Neutral Position (degrees)/1 -> Degrees to Radians/1
  DC to Rad/1(Position (rad)) -> Plus/1  "Position (rad)"
  Plus/1 -> Simulink-PS Converter/1  "Position (rad)"
  Degrees to Radians/1 -> Plus1/2, Plus/2
  PS-Simulink Converter/1 -> Plus1/1
  Plus1/1 -> Servo Position (rad)/1
  connections:
  PS-Simulink Converter/LConn1 -- Servomotor/RConn2
  Physical Art 2/RConn1 -- Servomotor/RConn1
  Servomotor/LConn1 -- Physical Art 1/RConn1
  Servomotor/LConn2 -- Simulink-PS Converter/RConn1

== system back_left_leg_assembly/Back Left Leg/Servomotor + Driver (Hip Joint X Axis)/Servomotor/DC to Rad ==
  DC (0 -->1) : Inport
  Bias2 : Bias  Bias=robot_conversions.DC_offset  SaturateOnIntegerOverflow=off
  Gain2 : Gain  Gain=robot_conversions.DC_to_rad
  Position (rad) : Outport
  wires:
  DC (0 -->1)/1 -> Bias2/1
  Bias2/1 -> Gain2/1
  Gain2/1 -> Position (rad)/1

== system back_left_leg_assembly/Back Left Leg/Servomotor + Driver (Hip Joint Y Axis)/Servomotor/DC to Rad ==
  DC (0 -->1) : Inport
  Bias2 : Bias  Bias=robot_conversions.DC_offset  SaturateOnIntegerOverflow=off
  Gain2 : Gain  Gain=robot_conversions.DC_to_rad
  Position (rad) : Outport
  wires:
  DC (0 -->1)/1 -> Bias2/1
  Bias2/1 -> Gain2/1
  Gain2/1 -> Position (rad)/1

== system back_left_leg_assembly/Back Left Leg/Left Leg Without Hip/Servomotor + Driver (Knee Joint Y Axis)/Servomotor/DC to Rad ==
  DC (0 -->1) : Inport
  Bias2 : Bias  Bias=robot_conversions.DC_offset  SaturateOnIntegerOverflow=off
  Gain2 : Gain  Gain=robot_conversions.DC_to_rad
  Position (rad) : Outport
  wires:
  DC (0 -->1)/1 -> Bias2/1
  Bias2/1 -> Gain2/1
  Gain2/1 -> Position (rad)/1
